simulink subsystem "balancing_active"  (R2021a)
settings: Solver=VariableStepAuto  StartTime=0.0  StopTime=10.0  RelTol=1e-3
libraries: fl_lib x30, ee_lib x10, nesl_utility x10
settings Model: Creator=DanielaDelliNoci  LastModifiedBy=Carlo Edoardo

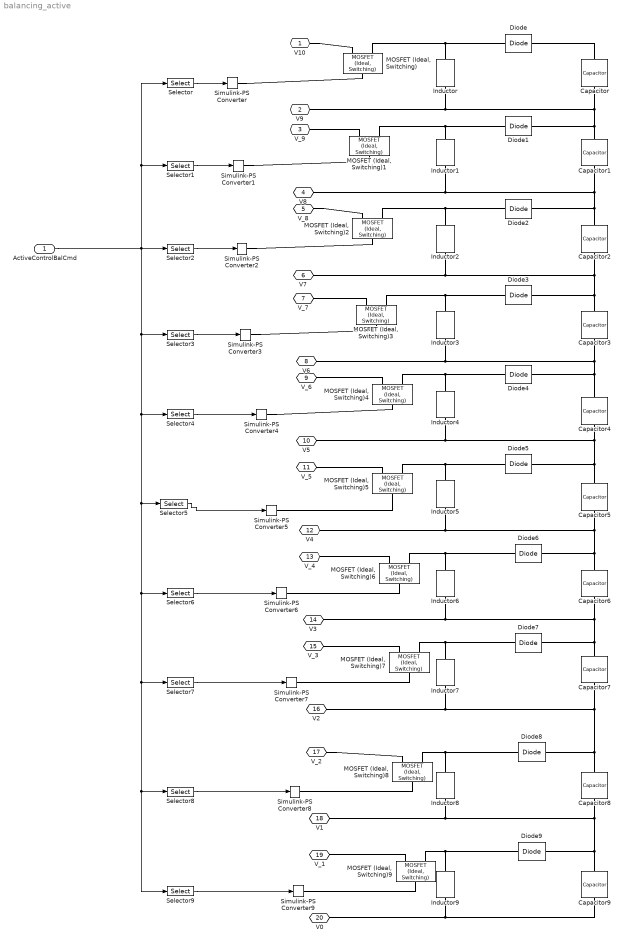
== system balancing_active ==
  ActiveControlBalCmd : Inport
  Capacitor{,1..9} (10 alike) : fl_lib/Electrical/Electrical Elements/Capacitor  c=1e-6 F  r=1e-6 Ohm  g=0 1/Ohm  i_specify=off  i_priority=None  i=0 A  i_nominal_specify=off  i_nominal_unit=A  i_nominal_value=1  v_specify=off  v_priority=None  v=0 V  v_nominal_specify=off  v_nominal_unit=V  v_nominal_value=1  vc_specify=off  vc_priority=High  vc=0 V  vc_nominal_specify=off  vc_nominal_unit=V  vc_nominal_value=1
  Diode{,1..9} (10 alike) : fl_lib/Electrical/Electrical Elements/Diode  Vf=0.6 V  Ron=0.3 Ohm  Goff=1e-8 1/Ohm  i_specify=off  i_priority=None  i=0 A  i_nominal_specify=off  i_nominal_unit=A  i_nominal_value=1  v_specify=off  v_priority=None  v=0 V  v_nominal_specify=off  v_nominal_unit=V  v_nominal_value=1
  Inductor{,1..9} (10 alike) : fl_lib/Electrical/Electrical Elements/Inductor  l=1e-6 H  r=0 Ohm  g=1e-9 1/Ohm  i_specify=off  i_priority=None  i=0 A  i_nominal_specify=off  i_nominal_unit=A  i_nominal_value=1  v_specify=off  v_priority=None  v=0 V  v_nominal_specify=off  v_nominal_unit=V  v_nominal_value=1  i_L_specify=off  i_L_priority=High  i_L=0 A  i_L_nominal_specify=off  i_L_nominal_unit=A  i_L_nominal_value=1
  MOSFET (Ideal, Switching){,1..9} (10 alike) : ee_lib/Semiconductors & Converters/MOSFET (Ideal, Switching)  Rds=0.01 Ohm  Goff=1e-6 1/Ohm  Vth=2 V  diode_param=ee.enum.converters.protectiondiode.none  diode_Vf=0.8 V  diode_Ron=0.001 Ohm  diode_Goff=1e-5 1/Ohm  diode_C=50e-9 F  diode_iRM=-235 A  diode_iF=300 A  diode_idot=-50 A/us  diode_trr_param=ee.enum.converters.diodetrr.trr_factor  diode_trr_factor=3  diode_trr=15 us  diode_Qrr=1500 s*uA  thermal_loss_option=ee.enum.converters.thermalLossOption.constantvalues  Von_data=[0, 1.1, 1.3, 1.45, 1.75, 2.25, 2.7; 0, 1, 1.15, 1.35, 1.7, 2.35, 3] V  Eon_data=[0, .29, 1.43, 2.86, 5.71, 13.14, 22.86; 0, .57, 2.63, 5.14, 10.29, 20.57, 30.29] * 1e-3 J  Eoff_data=[0, .21, 1.07, 2.14, 4.29, 9.86, 17.14; 0, .43, 1.97, 3.86, 7.71, 15.43, 22.71] * 1e-3 J  Tj=[298.15, 398.15] K  Iout_data=[0, 10, 50, 100, 200, 400, 600] A  Eon_scalar=22.86e-3 J  Eoff_scalar=17.14e-3 J  Voff=300 V  Iout_scalar=600 A  diodeModelType=ee.enum.converters.diodeModelType.pwl  diode_IfMat=[.07, .12, .19, 1.75, 4.24, 7.32, 11.2; .16, .3, .72, 2.14, 4.02, 6.35, 9.12] A  diode_TjVec=[25, 125] degC  diode_VfVec=[.5, .7, .9, 1.3, 1.7, 2.1, 2.5] V  thermal_network_parameterization=ee.enum.thermalNetworkTopology.external  Rth=[.03, .2] K/W  Rth_Foster=[.03, .2] K/W  thermal_mass_parameterization=ee.enum.thermalNetwork.timeconstant  thermal_mass=[3, 25] J/K  thermal_mass_Foster=[33, 50] J/K  thermal_time_constant=[.1, 5] s  thermal_time_constant_Foster=[1, 10] s  thermal_mass_initial_temperatures=[25, 25] degC  junction_thermal_mass=0.1 J/K  vT_specify=off  vT_priority=None  vT=0 V  vT_nominal_specify=off  vT_nominal_unit=V  vT_nominal_value=1  Qj_specify=off  Qj_priority=None  Qj=0 W  Qj_nominal_specify=off  Qj_nominal_unit=W  Qj_nominal_value=1  junction_temperature_specify=off  junction_temperature_priority=None  junction_temperature=25 degC  junction_temperature_nominal_specify=off  junction_temperature_nominal_unit=degC  junction_temperature_nominal_value=1
  Selector : Selector  InputPortWidth=10  IndexOptions=Index vector (dialog)  Indices=10  OutputSizes=1
  Selector1 : Selector  InputPortWidth=10  IndexOptions=Index vector (dialog)  Indices=9  OutputSizes=1
  Selector2 : Selector  InputPortWidth=10  IndexOptions=Index vector (dialog)  Indices=8  OutputSizes=1
  Selector3 : Selector  InputPortWidth=10  IndexOptions=Index vector (dialog)  Indices=7  OutputSizes=1
  Selector4 : Selector  InputPortWidth=10  IndexOptions=Index vector (dialog)  Indices=6  OutputSizes=1
  Selector5 : Selector  InputPortWidth=10  IndexOptions=Index vector (dialog)  Indices=5  OutputSizes=1
  Selector6 : Selector  InputPortWidth=10  IndexOptions=Index vector (dialog)  Indices=4  OutputSizes=1
  Selector7 : Selector  InputPortWidth=10  IndexOptions=Index vector (dialog)  Indices=3  OutputSizes=1
  Selector8 : Selector  InputPortWidth=10  IndexOptions=Index vector (dialog)  Indices=2  OutputSizes=1
  Selector9 : Selector  InputPortWidth=10  IndexOptions=Index vector (dialog)  Indices=1  OutputSizes=1
  Simulink-PS Converter{,1..9} (10 alike) : nesl_utility/Simulink-PS Converter  PhysicalDomain=network_engine_domain  SubClassName=ps_input  LeftPortType=input  RightPortType=output  PseudoPeriodic=off  Frequencies=[]  NoiseDistribution=none  NoiseParameters=[]  Unit=1  AffineConversion=off  FilteringAndDerivatives=provide  SimscapeFilterOrder=1  InputFilterTimeConstant=0.001  UdotUserProvided=0
      settings: SourceProductBaseCode=PW,SS
  V10 : PMIOPort  Side=Left
  V9 : PMIOPort  Port=2  Side=Left
  V_9 : PMIOPort  Port=3  Side=Left
  V8 : PMIOPort  Port=4  Side=Left
  V_8 : PMIOPort  Port=5  Side=Left
  V7 : PMIOPort  Port=6  Side=Left
  V_7 : PMIOPort  Port=7  Side=Left
  V6 : PMIOPort  Port=8  Side=Left
  V_6 : PMIOPort  Port=9  Side=Left
  V5 : PMIOPort  Port=10  Side=Left
  V_5 : PMIOPort  Port=11  Side=Left
  V4 : PMIOPort  Port=12  Side=Left
  V_4 : PMIOPort  Port=13  Side=Left
  V3 : PMIOPort  Port=14  Side=Left
  V_3 : PMIOPort  Port=15  Side=Left
  V2 : PMIOPort  Port=16  Side=Left
  V_2 : PMIOPort  Port=17  Side=Left
  V1 : PMIOPort  Port=18  Side=Left
  V_1 : PMIOPort  Port=19  Side=Left
  V0 : PMIOPort  Port=20  Side=Left
  wires:
  Selector2/1 -> Simulink-PS Converter2/1
  Selector6/1 -> Simulink-PS Converter6/1
  ActiveControlBalCmd/1 -> Selector2/1, Selector3/1, Selector4/1, Selector5/1, Selector6/1, Selector7/1, Selector8/1, Selector9/1, Selector1/1, Selector/1
  Selector5/1 -> Simulink-PS Converter5/1
  Selector/1 -> Simulink-PS Converter/1
  Selector3/1 -> Simulink-PS Converter3/1
  Selector9/1 -> Simulink-PS Converter9/1
  Selector8/1 -> Simulink-PS Converter8/1
  Selector1/1 -> Simulink-PS Converter1/1
  Selector4/1 -> Simulink-PS Converter4/1
  Selector7/1 -> Simulink-PS Converter7/1
  connections:
  Inductor1/LConn1 -- "MOSFET (Ideal, Switching)1"/RConn2 -- Diode1/RConn1
  Inductor3/LConn1 -- "MOSFET (Ideal, Switching)3"/RConn2 -- Diode3/RConn1
  Capacitor9/LConn1 -- Inductor9/RConn1 -- V0/RConn1
  Inductor8/LConn1 -- "MOSFET (Ideal, Switching)8"/RConn2 -- Diode8/RConn1
  Capacitor5/LConn1 -- Capacitor6/RConn1 -- Diode6/LConn1 -- Inductor5/RConn1 -- V4/RConn1
  Capacitor3/LConn1 -- Inductor3/RConn1 -- V6/RConn1 -- Capacitor4/RConn1 -- Diode4/LConn1
  Inductor4/LConn1 -- "MOSFET (Ideal, Switching)4"/RConn2 -- Diode4/RConn1
  Capacitor6/LConn1 -- Inductor6/RConn1 -- V3/RConn1 -- Capacitor7/RConn1 -- Diode7/LConn1
  Capacitor1/LConn1 -- Capacitor2/RConn1 -- Diode2/LConn1 -- Inductor1/RConn1 -- V8/RConn1
  Inductor2/LConn1 -- "MOSFET (Ideal, Switching)2"/RConn2 -- Diode2/RConn1
  Capacitor2/LConn1 -- Inductor2/RConn1 -- V7/RConn1 -- Capacitor3/RConn1 -- Diode3/LConn1
  Capacitor/LConn1 -- Capacitor1/RConn1 -- Diode1/LConn1 -- Inductor/RConn1 -- V9/RConn1
  Capacitor4/LConn1 -- Inductor4/RConn1 -- V5/RConn1 -- Capacitor5/RConn1 -- Diode5/LConn1
  Capacitor8/LConn1 -- Inductor8/RConn1 -- V1/RConn1 -- Diode9/LConn1 -- Capacitor9/RConn1
  Capacitor7/LConn1 -- Inductor7/RConn1 -- V2/RConn1 -- Capacitor8/RConn1 -- Diode8/LConn1
  Inductor/LConn1 -- Diode/RConn1 -- "MOSFET (Ideal, Switching)"/RConn2
  Inductor7/LConn1 -- "MOSFET (Ideal, Switching)7"/RConn2 -- Diode7/RConn1
  Inductor6/LConn1 -- "MOSFET (Ideal, Switching)6"/RConn2 -- Diode6/RConn1
  Inductor9/LConn1 -- Diode9/RConn1 -- "MOSFET (Ideal, Switching)9"/RConn2
  Inductor5/LConn1 -- "MOSFET (Ideal, Switching)5"/RConn2 -- Diode5/RConn1
  Diode/LConn1 -- Capacitor/RConn1
  V10/RConn1 -- "MOSFET (Ideal, Switching)"/RConn1
  Simulink-PS Converter1/RConn1 -- "MOSFET (Ideal, Switching)1"/LConn1
  V_3/RConn1 -- "MOSFET (Ideal, Switching)7"/RConn1
  V_1/RConn1 -- "MOSFET (Ideal, Switching)9"/RConn1
  V_6/RConn1 -- "MOSFET (Ideal, Switching)4"/RConn1
  Simulink-PS Converter2/RConn1 -- "MOSFET (Ideal, Switching)2"/LConn1
  V_7/RConn1 -- "MOSFET (Ideal, Switching)3"/RConn1
  "MOSFET (Ideal, Switching)6"/LConn1 -- Simulink-PS Converter6/RConn1
  Simulink-PS Converter4/RConn1 -- "MOSFET (Ideal, Switching)4"/LConn1
  V_2/RConn1 -- "MOSFET (Ideal, Switching)8"/RConn1
  Simulink-PS Converter5/RConn1 -- "MOSFET (Ideal, Switching)5"/LConn1
  V_8/RConn1 -- "MOSFET (Ideal, Switching)2"/RConn1
  "MOSFET (Ideal, Switching)7"/LConn1 -- Simulink-PS Converter7/RConn1
  Simulink-PS Converter3/RConn1 -- "MOSFET (Ideal, Switching)3"/LConn1
  "MOSFET (Ideal, Switching)8"/LConn1 -- Simulink-PS Converter8/RConn1
  V_9/RConn1 -- "MOSFET (Ideal, Switching)1"/RConn1
  Simulink-PS Converter/RConn1 -- "MOSFET (Ideal, Switching)"/LConn1
  "MOSFET (Ideal, Switching)9"/LConn1 -- Simulink-PS Converter9/RConn1
  V_4/RConn1 -- "MOSFET (Ideal, Switching)6"/RConn1
  V_5/RConn1 -- "MOSFET (Ideal, Switching)5"/RConn1
